simulink model "SimulinkSampleMotorJointMode"  (R2023b)
settings: Solver=VariableStepAuto  StartTime=0.0  StopTime=30  RelTol=1e-3
libraries: instrumentseriallib x5
settings Model: Creator=go_71  LastModifiedBy=go_71
settings SolverCC: AlgebraicLoopSolver=TrustRegion
settings DataIOCC: ReturnWorkspaceOutputs=off
settings DebuggingCC: UnconnectedInputMsg=warning  UnconnectedOutputMsg=warning  UnconnectedLineMsg=warning  ArithmeticOperatorsInVariantConditions=warning
settings ModelReferenceCC: EnableRefExpFcnMdlSchedulingChecks=on
settings SFSimCC: SimUseLocalCustomCode=off  CustomCodeUndefinedFunction=UseInterfaceOnly
settings RTWCC: RTWUseLocalCustomCode=off

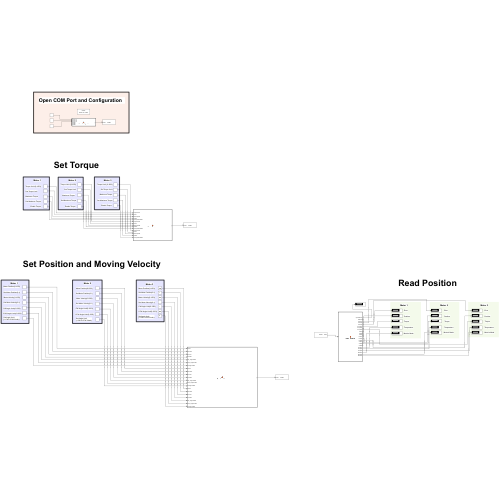
[thumbnail: Simulink's stored preview of the top-level diagram]
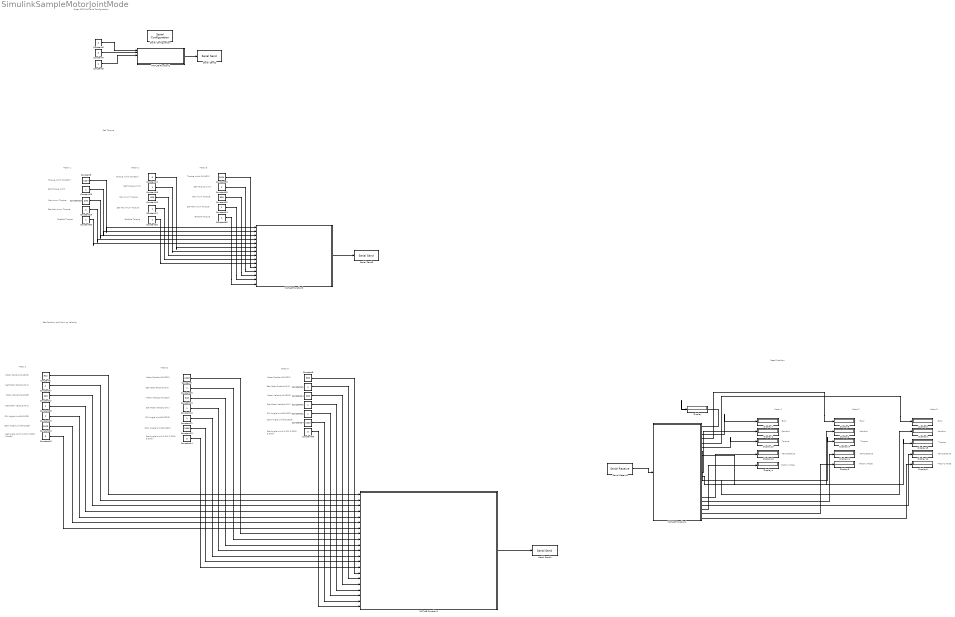
== system SimulinkSampleMotorJointMode ==
  note: Motor 1
  note: Motor 3
  note: Motor 2
  note: Motor Position(0-1023)
  note: Set Motor Position(0-1)
  note: Motor Velocity(0-1023)
  note: Set Motor Velocity(0-1)
  note: CW Angle Limit(0-1023)
  note: CCW Angle Limit(0-1023)
  note: Set Angle Limit
      | (1:CW 2:CCW 3:both)
  note: CCW Angle Limit(0-1023)
  note: Motor Position(0-1023)
  note: Set Motor Velocity(0-1)
  note: CW Angle Limit(0-1023)
  note: Motor Velocity(0-1023)
  note: Set Motor Position(0-1)
  note: CCW Angle Limit(0-1023)
  note: Motor Position(0-1023)
  note: Set Motor Velocity(0-1)
  note: CW Angle Limit(0-1023)
  note: Motor Velocity(0-1023)
  note: Set Motor Position(0-1)
  note: Set Angle Limit
      | (1:CW 2:CCW 3:both)
  note: Set Angle Limit
      | (1:CW 2:CCW 3:both)
  note: Motor 1
  note: Error
  note: Set Position and Moving Velocity
  note: Position
  note: Temperature
  note: Motor's Mode
  note: Motor's Mode
  note: Position
  note: Temperature
  note: Error
  note: Motor 2
  note: Error
  note: Position
  note: Temperature
  note: Motor's Mode
  note: Motor 3
  note: Read Position
  note: Open COM Port and Configuration
  note: Motor 1
  note: Torque Limit (0-1023)
  note: Set Torque Limit
  note: Maximum Torque
  note: Set Maximum Torque
  note: Enable Torque
  note: Torque Limit (0-1023)
  note: Enable Torque
  note: Set Torque Limit
  note: Maximum Torque
  note: Set Maximum Torque
  note: Motor 2
  note: Maximum Torque
  note: Set Maximum Torque
  note: Set Torque Limit
  note: Torque Limit (0-1023)
  note: Motor 3
  note: Enable Torque
  note: Set Torque
  note: Torque
  note: Torque
  note: Torque
  Constant10 : Constant  Value=500  SampleTime=1
  Constant11 : Constant  Value=0  SampleTime=1
  Constant12 : Constant  Value=100  SampleTime=1
  Constant13 : Constant  Value=300  SampleTime=1
  Constant14 : Constant  Value=250  SampleTime=1
  Constant18 : Constant  Value=200  SampleTime=1
  Constant{19,21..22,26..31,34..42} (18 alike) : Constant  SampleTime=1
  Constant20 : Constant  Value=1023  SampleTime=1
  Constant23 : Constant  Value=1000  SampleTime=1
  Constant24 : Constant  Value=1023  SampleTime=1
  Constant3 : Constant  Value=2  SampleTime=1
  Constant32 : Constant  Value=500  SampleTime=1
  Constant33 : Constant  Value=1024  SampleTime=1
  Constant4 : Constant  Value=2  SampleTime=1
  Constant43 : Constant  Value=3  SampleTime=1
  Constant44 : Constant  Value=3  SampleTime=1
  Constant45 : Constant  Value=3  SampleTime=1
  Constant5 : Constant  Value=2  SampleTime=1
  Constant6 : Constant  Value=512  SampleTime=1
  Constant7 : Constant  Value=1000  SampleTime=1
  Constant8 : Constant  Value=950  SampleTime=1
  Constant9 : Constant  Value=1024  SampleTime=1
  Display{,1..15} (16 alike) : Display
  MATLAB Function1 : MATLAB Function  Priority=2  TreatAsAtomicUnit=on
  MATLAB Function2 : MATLAB Function  Priority=1  TreatAsAtomicUnit=on  SystemSampleTime=1
  MATLAB Function3 : MATLAB Function  Priority=2  TreatAsAtomicUnit=on
  MATLAB Function4 : MATLAB Function  Priority=3  TreatAsAtomicUnit=on
  Serial Configuration : instrumentseriallib/Serial Configuration  Priority=-200000  PortSel=COM3  Port=COM3  ComPort=COM3  BaudRate=9600  DataBits=8  Parity=none  StopBits=1  ByteOrder=little-endian  FlowControl=none  Timeout=10  SimulateUsing=Interpreted execution  BlockInModel=on  aMode=1
  Serial Receive : instrumentseriallib/Serial Receive  PortSel=COM3  Port=COM3  ComPort=COM3  DataType=uint8  SaveDataType=uint8  ToggleHeader=off  Header=[]  ToggleTerminator=on  Terminator=<none>  CustomTerminator=[]  InputFormat=Column major  ToggleDataSize=on  DataSize="[64   1]"  EnableBlockingMode=on  ActionDataUnavailable=Output last received value  ActionWhenDataUnavailable=Output last received value  CustomValue=0  SampleTime=0.01  SimulateUsing=Interpreted execution  BlockInModel=on  aMode=1
  Serial Send1 : instrumentseriallib/Serial Send  PortSel=COM3  Port=COM3  ComPort=COM3  Header=[]  Terminator=<none>  CustomTerminator=[]  EnableBlockingMode=on  SimulateUsing=Interpreted execution  BlockInModel=on  aMode=1
  Serial Send2 : instrumentseriallib/Serial Send  PortSel=COM3  Port=COM3  ComPort=COM3  Header=[]  Terminator=<none>  CustomTerminator=[]  EnableBlockingMode=on  SimulateUsing=Interpreted execution  BlockInModel=on  aMode=1
  Serial Send3 : instrumentseriallib/Serial Send  PortSel=COM3  Port=COM3  ComPort=COM3  Header=[]  Terminator=<none>  CustomTerminator=[]  EnableBlockingMode=on  SimulateUsing=Interpreted execution  BlockInModel=on  aMode=1
  wires:
  Constant3/1 -> MATLAB Function2/1(mode_m1)
  Constant4/1 -> MATLAB Function2/2(mode_m2)
  Constant5/1 -> MATLAB Function2/3(mode_m3)
  Constant9/1 -> MATLAB Function3/1(TorqueLimM1)
  Constant30/1 -> MATLAB Function3/5(setTorqueEnableM1)
  Constant32/1 -> MATLAB Function3/13(MaxTorqueM3)
  Constant28/1 -> MATLAB Function3/7(setTL2)
  Constant27/1 -> MATLAB Function3/9(setMT2)
  Constant34/1 -> MATLAB Function3/14(setMT3)
  Constant18/1 -> MATLAB Function3/3(MaxTorqueM1)
  Constant31/1 -> MATLAB Function3/10(setTorqueEnableM2)
  Constant36/1 -> MATLAB Function3/15(setTorqueEnableM3)
  Constant11/1 -> MATLAB Function3/6(TorqueLimM2)
  Constant10/1 -> MATLAB Function3/8(MaxTorqueM2)
  Constant26/1 -> MATLAB Function3/2(setTL1)
  Constant29/1 -> MATLAB Function3/4(setMT1)
  Constant35/1 -> MATLAB Function3/12(setTL3)
  Constant33/1 -> MATLAB Function3/11(TorqueLimM3)
  MATLAB Function4/22(ModeM2) -> Display5/1
  MATLAB Function4/12(PosM1) -> Display1/1
  MATLAB Function4/4(ErrorM2) -> Display8/1
  Serial Receive/1 -> MATLAB Function4/1(u)
  MATLAB Function4/23(ModeM3) -> Display6/1
  MATLAB Function4/3(ErrorM1) -> Display7/1
  MATLAB Function4/13(PosM2) -> Display2/1
  MATLAB Function4/14(PosM3) -> Display3/1
  MATLAB Function4/5(ErrorM3) -> Display9/1
  MATLAB Function4/19(TempM2) -> Display11/1
  MATLAB Function4/20(TempM3) -> Display12/1
  MATLAB Function4/21(ModeM1) -> Display4/1
  MATLAB Function4/1(SystemMode) -> Display/1
  MATLAB Function4/18(TempM1) -> Display10/1
  Constant13/1 -> MATLAB Function1/10(MovVel2)
  Constant7/1 -> MATLAB Function1/8(PosM2)
  Constant23/1 -> MATLAB Function1/13(CCW_AngleLimitM2)
  Constant8/1 -> MATLAB Function1/15(PosM3)
  Constant24/1 -> MATLAB Function1/20(CCW_AngleLimitM3)
  Constant12/1 -> MATLAB Function1/3(MovVel1)
  Constant6/1 -> MATLAB Function1/1(PosM1)
  Constant21/1 -> MATLAB Function1/12(CW_AngleLimitM2)
  Constant40/1 -> MATLAB Function1/11(setVelM2)
  Constant43/1 -> MATLAB Function1/7(setAngleLimitM1)
  Constant39/1 -> MATLAB Function1/9(setPosM2)
  Constant38/1 -> MATLAB Function1/4(setVelM1)
  Constant14/1 -> MATLAB Function1/17(MovVel3)
  Constant42/1 -> MATLAB Function1/18(setVelM3)
  Constant20/1 -> MATLAB Function1/6(CCW_AngleLimitM1)
  MATLAB Function1/1(y) -> Serial Send1/1
  Constant45/1 -> MATLAB Function1/21(setAngleLimitM3)
  Constant37/1 -> MATLAB Function1/2(setPosM1)
  Constant44/1 -> MATLAB Function1/14(setAngleLimitM2)
  Constant22/1 -> MATLAB Function1/19(CW_AngleLimitM3)
  Constant41/1 -> MATLAB Function1/16(setPosM3)
  Constant19/1 -> MATLAB Function1/5(CW_AngleLimitM1)
  MATLAB Function2/1(y) -> Serial Send2/1
  MATLAB Function3/1(y) -> Serial Send3/1
  MATLAB Function4/7(TorqueM2) -> Display14/1
  MATLAB Function4/8(TorqueM3) -> Display15/1
  MATLAB Function4/6(TorqueM1) -> Display13/1

== matlab function SimulinkSampleMotorJointMode/MATLAB Function4 ==
  data: u input; SystemMode output; Datarate output; ErrorM1 output; ErrorM2 output; ErrorM3 output; TorqueM1 output double size=[16 1]; TorqueM2 output; TorqueM3 output; VelM1 output; VelM2 output; VelM3 output; PosM1 output; PosM2 output; PosM3 output; VoltM1 output; VoltM2 output; VoltM3 output; TempM1 output; TempM2 output; TempM3 output; ModeM1 output; ModeM2 output; ModeM3 output
function  [SystemMode,Datarate,ErrorM1,ErrorM2,ErrorM3,TorqueM1,TorqueM2,TorqueM3,VelM1,VelM2,VelM3,PosM1,PosM2,PosM3,VoltM1,VoltM2,VoltM3,TempM1,TempM2,TempM3, ModeM1,ModeM2,ModeM3] = ReadMotorsPacket(u)
%Read Motor Paquet
coder.extrinsic('extractBetween'); 
coder.extrinsic('str2num'); 

SystemMode = 0;
Datarate=0;
ErrorM1=0;
ErrorM2=0;
ErrorM3=0;
TorqueM1 = 0;
TorqueM2=0;
TorqueM3=0;
VelM1=0;
VelM2=0;
VelM3=0;
PosM1=0;
PosM2=0;
PosM3=0;
VoltM1=0;
VoltM2=0;
VoltM3=0;
TempM1=0;
TempM2=0;
TempM3=0;
ModeM1=0;
ModeM2=0;
ModeM3=0;

Utest = char(u);

SystemMode = double(uint8(u(2,1)));     %1:Motor   2:Encoder
Datarate = double(uint8(u(3,1)));       %0: Default 100 ms

ErrorM1=double(uint8(u(4,1)));
ErrorM2=double(uint8(u(5,1)));
ErrorM3=double(uint8(u(6,1)));

TorqueM1Aux = (typecast([uint8(u(7,1)) uint8(u(8,1))],'uint16'));
TorqueM2Aux = (typecast([uint8(u(9,1)) uint8(u(10,1))],'uint16'));
TorqueM3Aux = (typecast([uint8(u(11,1)) uint8(u(12,1))],'uint16'));

TorqueM1 =  double(bitand(TorqueM1Aux,uint16(1023)))*0.1;
TorqueM2 = double(bitand(TorqueM2Aux,uint16(1023)))*0.1;
TorqueM3 = double(bitand(TorqueM3Aux,uint16(1023)))*0.1;

VelM1Aux = typecast([uint8(u(13,1)) uint8(u(14,1))],'uint16');
VelM2Aux = typecast([uint8(u(15,1)) uint8(u(16,1))],'uint16');
VelM3Aux = typecast([uint8(u(17,1)) uint8(u(18,1))],'uint16');
VelM1 = double(bitand(VelM1Aux,uint16(1023)))*0.1;
VelM2 = double(bitand(VelM2Aux,uint16(1023)))*0.1;
VelM3 = double(bitand(VelM3Aux,uint16(1023)))*0.1;

PosM1Aux = typecast([uint8(u(19,1)) uint8(u(20,1))],'uint16');
PosM2Aux = typecast([uint8(u(21,1)) uint8(u(22,1))],'uint16');
PosM3Aux = typecast([uint8(u(23,1)) uint8(u(24,1))],'uint16');
PosM1 = double(PosM1Aux);
PosM2 = double(PosM2Aux);
PosM3 = double(PosM3Aux);

VoltM1 = double(uint8(u(25,1)))/10.0;
VoltM2 = double(uint8(u(26,1)))/10.0;
VoltM3 = double(uint8(u(27,1)))/10.0;

TempM1 = double(uint8(u(28,1)));
TempM2 = double(uint8(u(29,1)));
TempM3 = double(uint8(u(30,1)));

Mode  = de2bi(uint8(u(31,1)));
sm = size(Mode,2);
dif = 6-sm;
Mode6bits=[0 0 0 0 0 0 ];
for i=1:sm
    Mode6bits(i) = Mode(i);
end
for d=1:dif
    Mode6bits(sm+d)=0;
end

ModeM1Aux = bi2de(Mode6bits(1:2));
ModeM2Aux = bi2de(Mode6bits(3:4));
ModeM3Aux = bi2de(Mode6bits(5:6));
ModeM1 = double(ModeM1Aux); %1:Wheel 2:Joint
ModeM2 = double(ModeM2Aux);%1:Wheel 2:Joint
ModeM3 = double(ModeM3Aux);%1:Wheel 2:Joint

nop=1;

== matlab function SimulinkSampleMotorJointMode/MATLAB Function1 ==
  data: PosM1 input; setPosM1 input; MovVel1 input; setVelM1 input; CW_AngleLimitM1 input; CCW_AngleLimitM1 input; setAngleLimitM1 input; y output; PosM2 input; setPosM2 input; MovVel2 input; setVelM2 input; CW_AngleLimitM2 input; CCW_AngleLimitM2 input; setAngleLimitM2 input; PosM3 input; setPosM3 input; MovVel3 input; setVelM3 input; CW_AngleLimitM3 input; CCW_AngleLimitM3 input; setAngleLimitM3 input
function y = SetMotorsPosition(PosM1,setPosM1,MovVel1,setVelM1,CW_AngleLimitM1,CCW_AngleLimitM1,setAngleLimitM1,PosM2,setPosM2,MovVel2,setVelM2,CW_AngleLimitM2,CCW_AngleLimitM2,setAngleLimitM2,PosM3,setPosM3,MovVel3,setVelM3,CW_AngleLimitM3,CCW_AngleLimitM3,setAngleLimitM3)

coder.extrinsic('num2str'); 
Arr = uint8([1:32]);

%SET POSITION
set3= bitshift(setPosM3,2); 
set2= bitshift(setPosM2,1); 
setAux = bitor(set3,set2);
setPos = bitor(setPosM1,setAux);

inp= de2bi(PosM1,16);
LBits_arr = inp(1,1:8);
HBits_arr = inp(1,9:16);
LBitsM1 = bi2de(LBits_arr);
HBitsM1 = bi2de(HBits_arr);

inp2= de2bi(PosM2,16);
LBits_arr2 = inp2(1,1:8);
HBits_arr2 = inp2(1,9:16);
LBitsM2 = bi2de(LBits_arr2);
HBitsM2 = bi2de(HBits_arr2);

inp3= de2bi(PosM3,16);
LBits_arr3 = inp3(1,1:8);
HBits_arr3 = inp3(1,9:16);
LBitsM3 = bi2de(LBits_arr3);
HBitsM3 = bi2de(HBits_arr3);

%SET VELOCITY
setv3= bitshift(setVelM3,2); 
setv2= bitshift(setVelM2,1); 
setAux = bitor(setv3,setv2);
setVel = bitor(setVelM1,setAux);

inp= de2bi(MovVel1,16);
LBits_arr = inp(1,1:8);
HBits_arr = inp(1,9:16);
VLBitsM1 = bi2de(LBits_arr);
VHBitsM1 = bi2de(HBits_arr);
 
inp2= de2bi(MovVel2,16);
LBits_arr2 = inp2(1,1:8);
HBits_arr2 = inp2(1,9:16);
VLBitsM2 = bi2de(LBits_arr2);
VHBitsM2 = bi2de(HBits_arr2);

inp3= de2bi(MovVel3,16);
LBits_arr3 = inp3(1,1:8);
HBits_arr3 = inp3(1,9:16);
VLBitsM3 = bi2de(LBits_arr3);
VHBitsM3 = bi2de(HBits_arr3);

%ANGLE LIMIT CW AND CCW
setal3 = bitshift(setAngleLimitM3,4); 
setal2 = bitshift(setAngleLimitM2,2); 
setAux = bitor(setal3,setal2);
setAL  = bitor(setAngleLimitM1,setAux);

inp= de2bi(CW_AngleLimitM1,16);
LBits_arr = inp(1,1:8);
HBits_arr = inp(1,9:16);
ACW_LBitsM1 = bi2de(LBits_arr);
ACW_HBitsM1 = bi2de(HBits_arr);

inp= de2bi(CCW_AngleLimitM1,16);
LBits_arr = inp(1,1:8);
HBits_arr = inp(1,9:16);
ACCW_LBitsM1 = bi2de(LBits_arr);
ACCW_HBitsM1 = bi2de(HBits_arr);

inp= de2bi(CW_AngleLimitM2,16);
LBits_arr = inp(1,1:8);
HBits_arr = inp(1,9:16);
ACW_LBitsM2 = bi2de(LBits_arr);
ACW_HBitsM2 = bi2de(HBits_arr);

inp= de2bi(CCW_AngleLimitM2,16);
LBits_arr = inp(1,1:8);
HBits_arr = inp(1,9:16);
ACCW_LBitsM2 = bi2de(LBits_arr);
ACCW_HBitsM2 = bi2de(HBits_arr);

inp= de2bi(CW_AngleLimitM3,16);
LBits_arr = inp(1,1:8);
HBits_arr = inp(1,9:16);
ACW_LBitsM3 = bi2de(LBits_arr);
ACW_HBitsM3 = bi2de(HBits_arr);

inp= de2bi(CCW_AngleLimitM3,16);
LBits_arr = inp(1,1:8);
HBits_arr = inp(1,9:16);
ACCW_LBitsM3 = bi2de(LBits_arr);
ACCW_HBitsM3 = bi2de(HBits_arr);

Arr(1,1) =  122;
Arr(1,2) =  2;

Arr(1,3) =  setAL; %SET ANGLE LIMIT   0:0° 512:150°  a 1023:300°   
Arr(1,4) =  ACW_LBitsM1; %CW M1
Arr(1,5) =  ACW_HBitsM1; %CW M1
Arr(1,6) =  ACW_LBitsM2; %CW M2
Arr(1,7) =  ACW_HBitsM2; %CW M2
Arr(1,8) =  ACW_LBitsM3; %CW M3 
Arr(1,9) =  ACW_HBitsM3; %CW M3

Arr(1,10) =  ACCW_LBitsM1; %CCW M1
Arr(1,11) =  ACCW_HBitsM1; %CCW M1
Arr(1,12) =  ACCW_LBitsM2; %CCW M2
Arr(1,13) =  ACCW_HBitsM2; %CCW M2
Arr(1,14) =  ACCW_LBitsM3; %CCW M3
Arr(1,15) =  ACCW_HBitsM3; %CCW M3

Arr(1,16) =  setVel; %SET MOVING SPEED
Arr(1,17) =  VLBitsM1;
Arr(1,18) =  VHBitsM1;
Arr(1,19) =  VLBitsM2;
Arr(1,20) =  VHBitsM2;
Arr(1,21) =  VLBitsM3;
Arr(1,22) =  VHBitsM3;

Arr(1,23) =  setPos; %SET POSITION
Arr(1,24) =  LBitsM1;
Arr(1,25) =  HBitsM1;
Arr(1,26) =  LBitsM2;
Arr(1,27) =  HBitsM2;
Arr(1,28) =  LBitsM3;
Arr(1,29) =  HBitsM3;

Arr(1,30) =  0;
Arr(1,31) =  0; 
Arr(1,32) =  123;

y = Arr;

== matlab function SimulinkSampleMotorJointMode/MATLAB Function2 ==
  data: y output; mode_m1 input; mode_m2 input; mode_m3 input; LedM1 input; LedM2 input; LedM3 input
function y  = setMotorsConfiguration(mode_m1,mode_m2,mode_m3,LedM1,LedM2,LedM3)
%Paquete de configuracion del motor.
%mode_m1=1 -> Wheel
%mode_m1=2 -> Joint

s.init = 122;   %0x7A   122
s.mode = 3;  %3 Significa configuracion de motor.
s.set_mode_m1 = 48 ;   %0x31 = 49 = char '1'
s.set_mode_m2 = 48 ;   %0x31 = 49 = char '1'
s.set_mode_m3 = 48 ;   %0x31 = 49 = char '1'
s.mode_m1 = 49 ;  %49 = char '1' Wheel   50 = char '2' Joint
s.mode_m2 = 49 ;  %49 = char '1' Wheel   50 = char '2' Joint
s.mode_m3 = 49 ;  %49 = char '1' Wheel   50 = char '2' Joint

if mode_m1~=0
    s.set_mode_m1 = 49 ;   %0x31 = 49 = char '1'
    if mode_m1==1 %Mode Wheel
        s.mode_m1 = 49 ;  %49 = char '1' Wheel 
    elseif mode_m1==2  
        s.mode_m1 = 50 ;  %50 = char '2' Joint
    end
end

if mode_m2~=0
    s.set_mode_m2 = 49 ;   %0x31 = 49 = char '1'
    if mode_m2==1 %Mode Wheel
        s.mode_m2 = 49 ;  %49 = char '1' Wheel  
    elseif mode_m2==2  
        s.mode_m2 = 50 ;  %50 = char '2' Joint
    end
end

if mode_m3~=0
    s.set_mode_m3 = 49 ;   %0x31 = 49 = char '1'
    if mode_m3 == 1 %Mode Wheel
        s.mode_m3 = 49 ;  %49 = char '1' Wheel
    elseif mode_m3==2  
        s.mode_m3 = 50 ;  %50 = char '2' Joint
    end
end


s.set_id_m1 = 0 ;
s.set_id_m2 = 0 ;
s.set_id_m3 = 0 ;

s.id_m1 = 0;
s.id_m2 = 0;
s.id_m3 = 0;

LEDM1 = 48;
if LedM1 ==1
    LEDM1 =49;
end

LEDM2 = 48;
if LedM2 ==1
    LEDM2 =49;
end

LEDM3 = 48;
if LedM3 ==1
    LEDM3 =49;
end

s.turnon_led_m1 = LEDM1;  %48:0  49:1
s.turnon_led_m2 = LEDM2;
s.turnon_led_m3 = LEDM3;

s.not_used17 = 0;
s.not_used18 = 0;
s.not_used19 = 0;

s.not_used20 = 0;
s.not_used21 = 0;
s.not_used22 = 0;
s.not_used23 = 0;
s.not_used24 = 0;
s.not_used25 = 0;
s.not_used26 = 0;
s.not_used27 = 0;
s.not_used28 = 0;
s.not_used29 = 0;
s.not_used30 = 1;  %Thiss byte has to be 1. 
s.finish = 123;  %0X7B

ArrToSend = uint8([s.init ;s.mode ; s.set_mode_m1; s.set_mode_m2; s.set_mode_m3; s.mode_m1;s.mode_m2;s.mode_m3;s.set_id_m1;s.set_id_m2;s.set_id_m3;s.id_m1;s.id_m2;s.id_m3;s.turnon_led_m1;s.turnon_led_m2;s.turnon_led_m3;s.not_used17;s.not_used18;s.not_used19;s.not_used20;s.not_used21;s.not_used22;s.not_used23;s.not_used24;s.not_used25;s.not_used26;s.not_used27;s.not_used28;s.not_used29; s.not_used30;s.finish]);
nop=1;
y = ArrToSend;

== matlab function SimulinkSampleMotorJointMode/MATLAB Function3 ==
  data: TorqueLimM1 input; setTL1 input; MaxTorqueM1 input; setMT1 input; setTorqueEnableM1 input; TorqueLimM2 input; setTL2 input; MaxTorqueM2 input; setMT2 input; setTorqueEnableM2 input; y output; TorqueLimM3 input; setTL3 input; MaxTorqueM3 input; setMT3 input; setTorqueEnableM3 input
function y = SetMotorsTorqueLimit(TorqueLimM1,setTL1,MaxTorqueM1,setMT1,setTorqueEnableM1,   TorqueLimM2,setTL2,MaxTorqueM2,setMT2,setTorqueEnableM2, TorqueLimM3,setTL3,MaxTorqueM3,setMT3,setTorqueEnableM3)
% Write Packet 1

Arr = uint8([1:32]);
coder.extrinsic('num2str'); 

%TORQUE LIMIT
set3= bitshift(setTL3,2); 
set2= bitshift(setTL2,1); 
setAux = bitor(set3,set2);
setTL = bitor(setTL1,setAux);

inp= de2bi(TorqueLimM1,16);
LBits_arr = inp(1,1:8);
HBits_arr = inp(1,9:16);
TL_LBitsM1 = bi2de(LBits_arr);
TL_HBitsM1 = bi2de(HBits_arr);
 
inp2= de2bi(TorqueLimM2,16);
LBits_arr2 = inp2(1,1:8);
HBits_arr2 = inp2(1,9:16);
TL_LBitsM2 = bi2de(LBits_arr2);
TL_HBitsM2 = bi2de(HBits_arr2);

inp3= de2bi(TorqueLimM3,16);
LBits_arr3 = inp3(1,1:8);
HBits_arr3 = inp3(1,9:16);
TL_LBitsM3 = bi2de(LBits_arr3);
TL_HBitsM3 = bi2de(HBits_arr3);

%MAX TORQUE
setmt3= bitshift(setMT3,2); 
setmt2= bitshift(setMT2,1); 
setmtAux = bitor(setmt3,setmt2);
setMT = bitor(setMT1,setmtAux);
nop=1;

inp= de2bi(MaxTorqueM1,16);
LBits_arr = inp(1,1:8);
HBits_arr = inp(1,9:16);
MT_LBitsM1 = bi2de(LBits_arr);
MT_HBitsM1 = bi2de(HBits_arr);

inp2= de2bi(MaxTorqueM2,16);
LBits_arr2 = inp2(1,1:8);
HBits_arr2 = inp2(1,9:16);
MT_LBitsM2 = bi2de(LBits_arr2);
MT_HBitsM2 = bi2de(HBits_arr2);

inp3= de2bi(MaxTorqueM3,16);
LBits_arr3 = inp3(1,1:8);
HBits_arr3 = inp3(1,9:16);
MT_LBitsM3 = bi2de(LBits_arr3);
MT_HBitsM3 = bi2de(HBits_arr3);

%Set TorqueENABLE
sette3= bitshift(setTorqueEnableM3,2); 
sette2= bitshift(setTorqueEnableM2,1); 
setmtAux = bitor(sette3,sette2);
setTorqueEnable = bitor(setTorqueEnableM1,setmtAux);

Arr(1,1) =  122;
Arr(1,2) =  1;
Arr(1,3) =  0;  % CONFIG DATA RATE
Arr(1,4) =  0;  % DATA RATE

Arr(1,5) =  setTorqueEnable;    %Torque Enable  %1-7

Arr(1,6) =  setTL;%Set Torque Limit
Arr(1,7) = TL_LBitsM1;
Arr(1,8) = TL_HBitsM1;
Arr(1,9) = TL_LBitsM2;
Arr(1,10) =TL_HBitsM2; 
Arr(1,11) = TL_LBitsM3;
Arr(1,12) = TL_HBitsM3;

Arr(1,13) =  setMT; %Set Torque Max 
Arr(1,14) =  MT_LBitsM1;
Arr(1,15) =  MT_HBitsM1;
Arr(1,16) =  MT_LBitsM2;
Arr(1,17) =  MT_HBitsM2;
Arr(1,18) =  MT_LBitsM3;
Arr(1,19) =  MT_HBitsM3;

Arr(1,20) =  0;
Arr(1,21) =  0;
Arr(1,22) =  0;
Arr(1,23) =  0;
Arr(1,24) =  0;
Arr(1,25) =  0;
Arr(1,26) =  0;
Arr(1,27) =  0;
Arr(1,28) =  0;
Arr(1,29) =  0;
Arr(1,30) =  0;

Arr(1,31) =  1;
Arr(1,32) =  123;

y = Arr;
